simulink model "GainScheduling"  (R2018b)
settings: Solver=VariableStepAuto  StartTime=0.0  StopTime=100  RelTol=1e-3
values from neighbouring files (symbols this model uses):
  A = [0 1; 2 -1]    [PolePlacement.m]
  B = [1; 0]    [PolePlacement.m]
  C = [1 0]    [PolePlacement.m]
  K = place(A, B, P)    [PolePlacement.m]
settings Model: Creator=Alex  LastModifiedBy=Alex

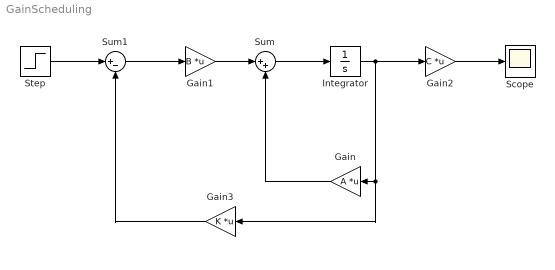
== system GainScheduling ==
  Gain : Gain  Gain=A  Multiplication=Matrix(K*u)
  Gain1 : Gain  Gain=B  Multiplication=Matrix(K*u)
  Gain2 : Gain  Gain=C  Multiplication=Matrix(K*u)
  Gain3 : Gain  Gain=K  Multiplication=Matrix(K*u)
  Integrator : Integrator
  Scope : Scope
  Step : Step  Time=0  SampleTime=0
  Sum : Sum  Inputs=|++
  Sum1 : Sum  Inputs=|+-
  wires:
  Integrator/1 -> Gain2/1, Gain3/1, Gain/1
  Gain/1 -> Sum/2
  Sum/1 -> Integrator/1
  Gain1/1 -> Sum/1
  Sum1/1 -> Gain1/1
  Gain3/1 -> Sum1/2
  Step/1 -> Sum1/1
  Gain2/1 -> Scope/1
